simulink model "SallenKeyFilter"  (R2020b)
settings: Solver=VariableStepAuto  StartTime=0.0  StopTime=10.0  RelTol=1e-3
libraries: fl_lib x9, nesl_utility x3, ee_lib x1
settings Model: Creator=Miodrag Bolic  LastModifiedBy=bolic
settings DataIOCC: ReturnWorkspaceOutputs=off
settings DebuggingCC: ArithmeticOperatorsInVariantConditions=warning
settings SFSimCC: CustomCodeUndefinedFunction=UseInterfaceOnly

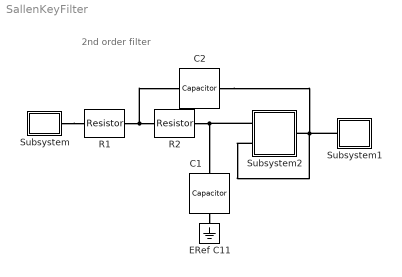
== system SallenKeyFilter ==
  note: 2nd order filter
  C1 : fl_lib/Electrical/Electrical Elements/Capacitor  c=100 nF  r=0 Ohm  g=0 1/Ohm  i_specify=off  i_priority=High  i=0 A  i_nominal_specify=off  i_nominal_unit=A  i_nominal_value=1  v_specify=off  v_priority=High  v=0 V  v_nominal_specify=off  v_nominal_unit=V  v_nominal_value=1  vc_specify=off  vc_priority=High  vc=0 V  vc_nominal_specify=off  vc_nominal_unit=V  vc_nominal_value=1
      settings: AttributesFormatString=%<c> %<c_unit>  SourceProductName=Foundation Library
  C2 : fl_lib/Electrical/Electrical Elements/Capacitor  c=200 nF  r=0 Ohm  g=0 1/Ohm  i_specify=off  i_priority=High  i=0 A  i_nominal_specify=off  i_nominal_unit=A  i_nominal_value=1  v_specify=off  v_priority=High  v=0 V  v_nominal_specify=off  v_nominal_unit=V  v_nominal_value=1  vc_specify=off  vc_priority=High  vc=0 V  vc_nominal_specify=off  vc_nominal_unit=V  vc_nominal_value=1
      settings: AttributesFormatString=%<c> %<c_unit>  SourceProductName=Foundation Library
  ERef C11 : fl_lib/Electrical/Electrical Elements/Electrical Reference
      settings: SourceProductName=Foundation Library
  R1 : fl_lib/Electrical/Electrical Elements/Resistor  R=69 kOhm  i_specify=off  i_priority=High  i=0 A  i_nominal_specify=off  i_nominal_unit=A  i_nominal_value=1  v_specify=off  v_priority=High  v=0 V  v_nominal_specify=off  v_nominal_unit=V  v_nominal_value=1
      settings: AttributesFormatString=%<R> %<R_unit>  SourceProductName=Foundation Library
  R2 : fl_lib/Electrical/Electrical Elements/Resistor  R=69 kOhm  i_specify=off  i_priority=High  i=0 A  i_nominal_specify=off  i_nominal_unit=A  i_nominal_value=1  v_specify=off  v_priority=High  v=0 V  v_nominal_specify=off  v_nominal_unit=V  v_nominal_value=1
      settings: AttributesFormatString=%<R> %<R_unit>  SourceProductName=Foundation Library
  Subsystem : Subsystem
      mask Display: disp('Vin')
  Subsystem1 : Subsystem
      mask Display: disp('Vo')
  Subsystem2 : Subsystem
      mask Display: image('op_amp_plus_up.png')
  connections:
  R2/LConn1 -- R1/RConn1 -- C2/LConn1
  C2/RConn1 -- Subsystem2/LConn2 -- Subsystem1/LConn1 -- Subsystem2/RConn1
  R2/RConn1 -- Subsystem2/LConn1 -- C1/LConn1
  C1/RConn1 -- ERef C11/LConn1
  Subsystem/RConn1 -- R1/LConn1

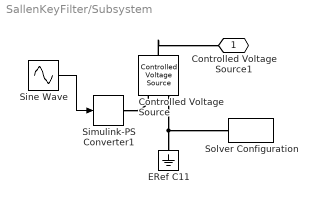
== system SallenKeyFilter/Subsystem ==
  Controlled Voltage Source : fl_lib/Electrical/Electrical Sources/Controlled Voltage Source
  ERef C11 : fl_lib/Electrical/Electrical Elements/Electrical Reference
      settings: SourceProductName=Foundation Library
  Simulink-PS Converter1 : nesl_utility/Simulink-PS Converter  PhysicalDomain=network_engine_domain  SubClassName=ps_input  LeftPortType=input  RightPortType=output  PseudoPeriodic=off  Frequencies=[]  NoiseDistribution=none  NoiseParameters=[]  Unit=V  AffineConversion=off  FilteringAndDerivatives=zero  SimscapeFilterOrder=1  InputFilterTimeConstant=.001  UdotUserProvided=0
  Sine Wave : Sin  Frequency=2*pi/4  SampleTime=0
  Solver Configuration : nesl_utility/Solver Configuration  PhysicalDomain=network_engine_domain  SubClassName=solver  LeftPortType=input  RightPortType=generic  Tones=[]  Harmonics=[]  SimulateNoise=off  Profile=off  UseLocalSampling=off  EnableSwitchedLinearOptims=on  FrequencyDomain=off  UseCCode=off  RelTol=0.001  AbsTol=1e-06  MinStep=1e-09  ToWorkspace=off  RevertToSquareIcSolve=off  NumHomotopyIterations=100  PhasorMode=off  PhasorModeNumHarmonics=1  DoDC=off  ResidualTolerance=1e-9  UseLocalSolver=off  LocalSolverChoice=NE_BACKWARD_EULER_ADVANCER  LocalSolverSampleTime=1e-6  DoFixedCost=off  MaxNonlinIter=3  MaxModeIter=2  ComputeImpulses=off  ImpulseIterations=2  LinearAlgebra=auto  EquationFormulation=NE_TIME_EF  DelaysMemoryBudget=1024  AutomaticFiltering=on  FilteringTimeConstant=0.001  PartitionStorageMethod=AS_NEEDED  PartitionMemoryBudget=1024  PartitionMethod=FAST
  Controlled Voltage Source1 : PMIOPort  Side=Right
  wires:
  Sine Wave/1 -> Simulink-PS Converter1/1
  connections:
  Simulink-PS Converter1/RConn1 -- Controlled Voltage Source/RConn1
  Controlled Voltage Source/LConn1 -- Controlled Voltage Source1/RConn1
  Controlled Voltage Source/RConn2 -- Solver Configuration/RConn1 -- ERef C11/LConn1

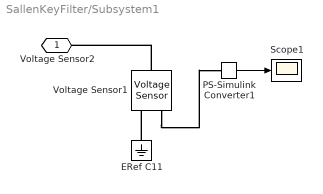
== system SallenKeyFilter/Subsystem1 ==
  " Scope1" : Scope
  ERef C11 : fl_lib/Electrical/Electrical Elements/Electrical Reference
      settings: SourceProductName=Foundation Library
  PS-Simulink Converter1 : nesl_utility/PS-Simulink Converter  PhysicalDomain=network_engine_domain  SubClassName=ps_output  LeftPortType=input  RightPortType=output  PseudoPeriodic=off  Frequencies=[]  Unit=1  AffineConversion=off
  Voltage Sensor1 : fl_lib/Electrical/Electrical Sensors/Voltage Sensor
  Voltage Sensor2 : PMIOPort  Side=Left
  wires:
  PS-Simulink Converter1/1 -> " Scope1"/1
  connections:
  Voltage Sensor1/LConn1 -- Voltage Sensor2/RConn1
  Voltage Sensor1/RConn1 -- PS-Simulink Converter1/LConn1
  ERef C11/LConn1 -- Voltage Sensor1/RConn2

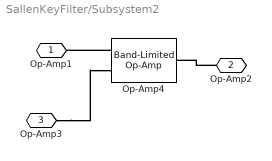
== system SallenKeyFilter/Subsystem2 ==
  Op-Amp4 : ee_lib/Integrated Circuits/Band-Limited Op-Amp  A=50000  Rin=6e+6 Ohm  Rout=100 Ohm  Vmin=-15 V  Vmax=15 V  Vdotmax=0.7e6 V/s  f=1.5e+6 Hz  V0=0 V
      settings: SourceProductBaseCode=PS
  Op-Amp1 : PMIOPort  Side=Left
  Op-Amp2 : PMIOPort  Port=2  Side=Right
  Op-Amp3 : PMIOPort  Port=3  Side=Left
  connections:
  Op-Amp4/LConn1 -- Op-Amp1/RConn1
  Op-Amp3/RConn1 -- Op-Amp4/LConn2
  Op-Amp2/RConn1 -- Op-Amp4/RConn1
